simulink model "Models"  (R2020a)
settings: Solver=VariableStepAuto  StartTime=0.0  StopTime=tFinal  MaxStep=tStepMax  RelTol=1e-3
values from neighbouring files (symbols this model uses):
  c = 0.5    [init.m]
  g = 10    [init.m]
  L = 1    [init.m]
  m = 1    [init.m]
  theta0 = 0*pi/180    (= 0)    [init.m]
  thetadot0 = 0    [init.m]
settings Model: Creator=hussein  LastModifiedBy=hussein

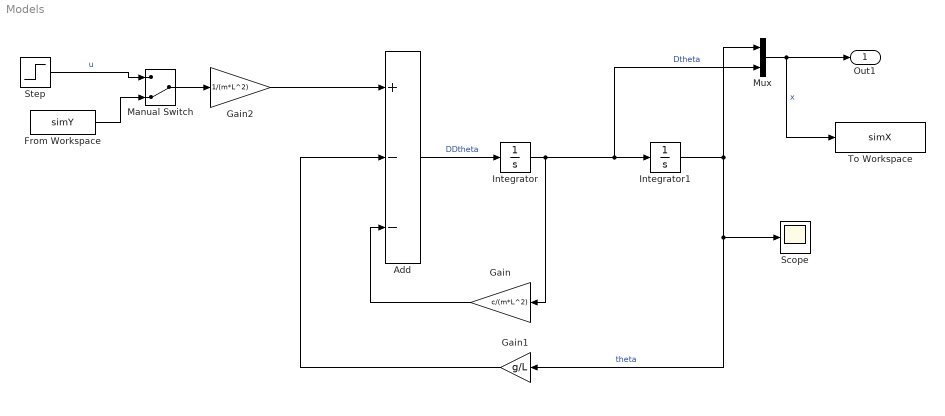
== system Models ==
  Add : Sum  Inputs=+--
  From Workspace : FromWorkspace  VariableName=simY
  Gain : Gain  Gain=c/(m*L^2)
  Gain1 : Gain  Gain=g/L
  Gain2 : Gain  Gain=1/(m*L^2)
  Integrator : Integrator  InitialCondition=thetadot0
  Integrator1 : Integrator  InitialCondition=theta0
  Manual Switch : ManualSwitch  CurrentSetting=0
  Mux : Mux  Inputs=2
  Scope : Scope
  Step : Step  Time=10  SampleTime=0
  To Workspace : ToWorkspace  VariableName=simX  SaveFormat=Timeseries  SampleTime=-1
  Out1 : Outport
  wires:
  Step/1 -> Manual Switch/1  "u"
  Add/1 -> Integrator/1  "DDtheta"
  Integrator/1 -> Gain/1, Mux/2, Integrator1/1  "Dtheta"
  Gain/1 -> Add/3
  Integrator1/1 -> Mux/1, Gain1/1, Scope/1  "theta"
  Gain1/1 -> Add/2
  Gain2/1 -> Add/1
  Mux/1 -> To Workspace/1, Out1/1  "x"
  Manual Switch/1 -> Gain2/1
  From Workspace/1 -> Manual Switch/2
